simulink model "rf"  (R2023b)
settings: Solver=VariableStepAuto  StartTime=0.0  StopTime=2000  RelTol=1e-3
libraries: commchan3 x1, commdigbbndpm3 x1, commrandsrc3 x1, eeGeneralControl x1
settings Model: Creator=HRama  LastModifiedBy=HRama

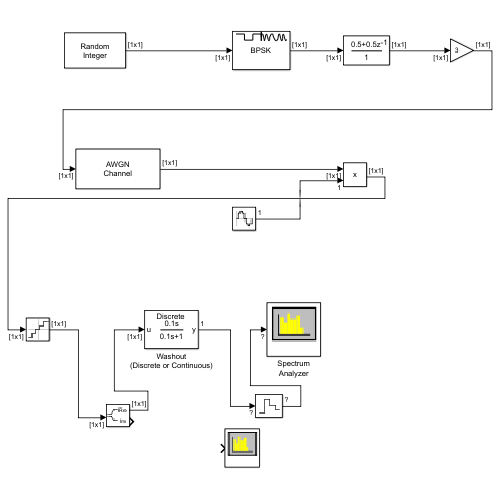
[thumbnail: Simulink's stored preview of the top-level diagram]
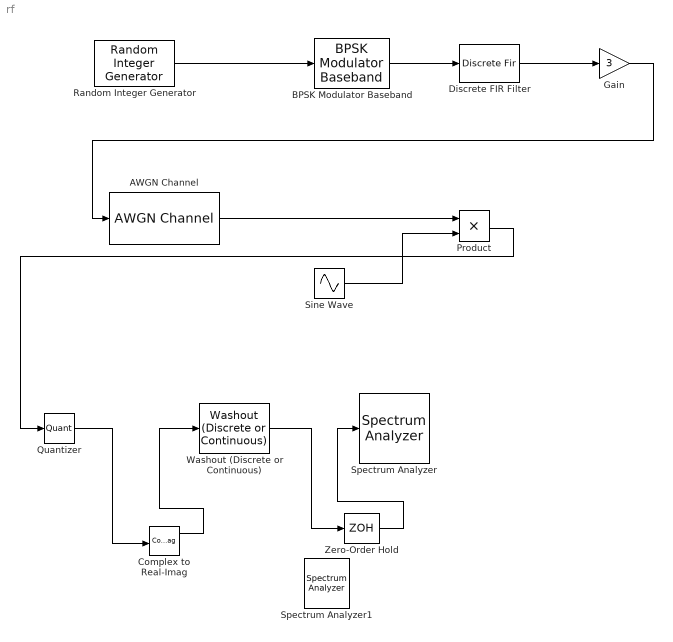
== system rf ==
  AWGN Channel : commchan3/AWGN Channel  LegacyMode=off  NoiseMethod="Signal to noise ratio  (SNR)"  noiseMode="Signal to noise ratio  (SNR)"  EbNo=10  EsNo=10  SNR=10  BitsPerSymbol=1  SignalPower=1  SamplesPerSymbol=1  SymbolPeriod=1  VarianceSource=Parameter  Variance=1  RandomStream=Global stream  Seed=67  SimulateUsing=Code generation
  BPSK Modulator Baseband : commdigbbndpm3/BPSK Modulator Baseband  Ph=0  outDtype=double  outWordLen=16  outUDDataType=sfix(16)  outFracLenMode=Best precision  outFracLen=15  outDataTypeStr=double  outLastDataTypeStr=double
  Complex to Real-Imag : ComplexToRealImag
  Discrete FIR Filter : DiscreteFir
  Gain : Gain  Gain=3
  Product : Product
  Quantizer : Quantizer
  Random Integer Generator : commrandsrc3/Random Integer Generator  SetSize=2  SeedSource=Auto  Seed=0  SampleTime=1  SamplesPerFrame=1  OutputDataType=double  SimulateUsing=Interpreted execution
  Sine Wave : Sin  Phase=2*pi  SampleTime=0.025
  Spectrum Analyzer : SpectrumAnalyzer  Tag=simrfV2util1/Spectrum Analyzer  WindowPosition=[1.000000,49.000000,1536.000000,889.000000,]  ScopeFrameLocation=window  ViewType=Spectrum and spectrogram  Method=Welch  Span=1  StartFrequency=-0.5  StopFrequency=0.5  AveragingMethod=Exponential  YLimits=[5.9206,38.9482]  ColorLimits=[5.9206,38.9482]  ShowLegend=on  SelectedToolstripTab=spectrumAnalyzerToolstrip.spectralMaskTab
  Spectrum Analyzer1 : SpectrumAnalyzer  WindowPosition=[368.000000,230.000000,800.000000,500.000000,]  ScopeFrameLocation=window  SampleRateSource=Property  SampleRate=44.1e3  PlotAsTwoSidedSpectrum=off  FrequencyScale=Log  FrequencySpan=Start and stop frequencies  StartFrequency=20  StopFrequency=20e3
  Washout (Discrete or Continuous) : eeGeneralControl/Washout (Discrete or Continuous)  T=0.1  init_option=Inherited from block input  x0=0  Ts=-1
      settings: LibrarySourceBlock=|
      | ee_sl_lib/General Control/Washout
      | (Discrete or Continuous)
  Zero-Order Hold : ZeroOrderHold  SampleTime=-1
  wires:
  Random Integer Generator/1 -> BPSK Modulator Baseband/1
  BPSK Modulator Baseband/1 -> Discrete FIR Filter/1
  Discrete FIR Filter/1 -> Gain/1
  AWGN Channel/1 -> Product/1
  Sine Wave/1 -> Product/2
  Gain/1 -> AWGN Channel/1
  Product/1 -> Quantizer/1
  Quantizer/1 -> Complex to Real-Imag/1
  Complex to Real-Imag/1 -> Washout (Discrete or Continuous)/1
  Zero-Order Hold/1 -> Spectrum Analyzer/1
  Washout (Discrete or Continuous)/1 -> Zero-Order Hold/1
